simulink model "PieroCinematica"  (R2022b)
settings: Solver=VariableStepAuto  StartTime=0.0  StopTime=10.0  RelTol=1e-3
settings Model: Creator=David  LastModifiedBy=David

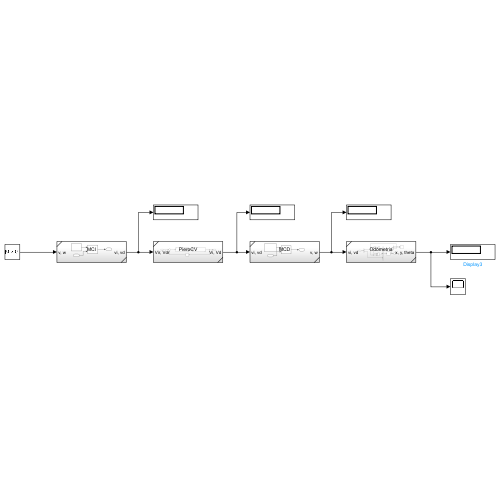
[thumbnail: Simulink's stored preview of the top-level diagram]
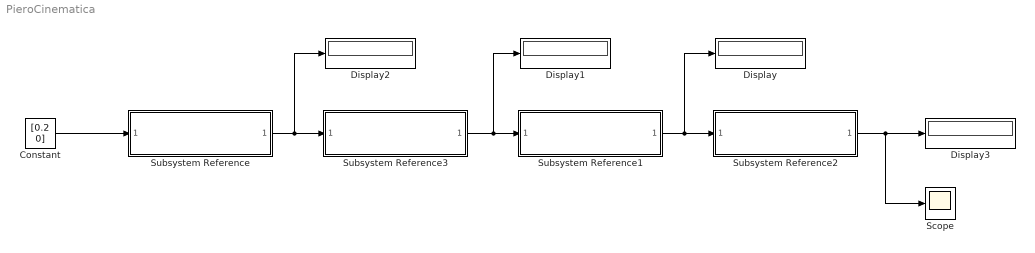
== system PieroCinematica ==
  Constant : Constant  Value=[0.2 0]
  Display{,1..3} (4 alike) : Display
  Scope : Scope
  Subsystem Reference : Subsystem  ReferencedSubsystem=MCI
  Subsystem Reference1 : Subsystem  ReferencedSubsystem=MCD
  Subsystem Reference2 : Subsystem  ReferencedSubsystem=Odometria
  Subsystem Reference3 : Subsystem  ReferencedSubsystem=PieroCV
  wires:
  Subsystem Reference1/1 -> Display/1, Subsystem Reference2/1
  Subsystem Reference/1 -> Display2/1, Subsystem Reference3/1
  Subsystem Reference3/1 -> Display1/1, Subsystem Reference1/1
  Constant/1 -> Subsystem Reference/1
  Subsystem Reference2/1 -> Scope/1, Display3/1
